simulink model "FM"  (R2021b)
settings: Solver=VariableStepAuto  StartTime=0.0  StopTime=10  MaxStep=0.05  RelTol=1e-3
libraries: commanapbnd3 x1
settings Model: Creator=USER  LastModifiedBy=USER

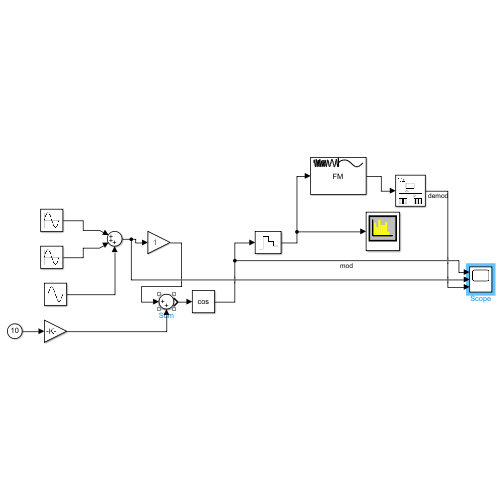
[thumbnail: Simulink's stored preview of the top-level diagram]
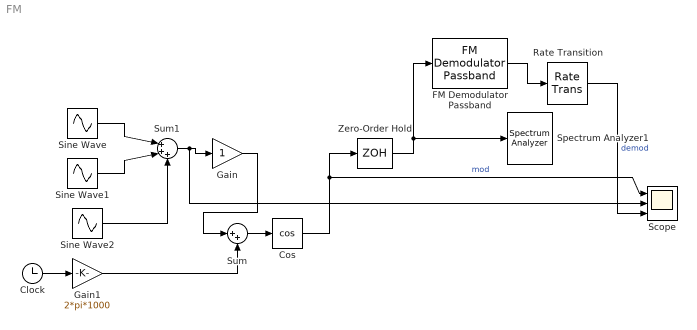
== system FM ==
  Clock : Clock
  Cos : Trigonometry  Operator=cos
  FM Demodulator Passband : commanapbnd3/FM Demodulator Passband  Fc=1000  Ph=0  Kc=500  Ho=100
      settings: SourceProductBaseCode=CM
  Gain : Gain
  Gain1 : Gain  Gain=2*pi*1000
  Rate Transition : RateTransition
  Scope : Scope  NumInputPorts=3
  Sine Wave : Sin  Frequency=2 * pi * 100  SampleTime=0
  Sine Wave1 : Sin  Frequency=2 * pi * 80  SampleTime=0
  Sine Wave2 : Sin  Frequency=2 * pi * 60  SampleTime=0
  Spectrum Analyzer1 : SpectrumAnalyzer
  Sum : Sum  Inputs=|++
  Sum1 : Sum  Inputs=|+++
  Zero-Order Hold : ZeroOrderHold  SampleTime=1e-4
  wires:
  Rate Transition/1 -> Scope/3  "demod"
  Cos/1 -> Zero-Order Hold/1, Scope/1  "mod"
  Gain1/1 -> Sum/2
  Clock/1 -> Gain1/1
  Sum/1 -> Cos/1
  Zero-Order Hold/1 -> FM Demodulator Passband/1, Spectrum Analyzer1/1
  FM Demodulator Passband/1 -> Rate Transition/1
  Sine Wave/1 -> Sum1/1
  Gain/1 -> Sum/1
  Sum1/1 -> Scope/2, Gain/1
  Sine Wave1/1 -> Sum1/2
  Sine Wave2/1 -> Sum1/3
